simulink model "Lab4_1simulink"  (R2024b)
settings: Solver=ode45  StartTime=0.0  StopTime=t_sim  MaxStep=0.01*Ts  MinStep=0.001*Ts  RelTol=1e-3
values from neighbouring files (symbols this model uses):
  C = [1 0]    [Lab_Practice_4_1.m]
  K = dlqr(Ad, Bd, Q,R)    [Lab_Practice_4_1.m]
  Ts = 0.05    [Lab_Practice_4_1.m]
  x0 = [0.8;0]    [Lab_Practice_4_1.m]
libraries: cstblocks x1
settings Model: Creator=filoz  LastModifiedBy=filoz
settings SolverCC: InitialStep=0.001*Ts

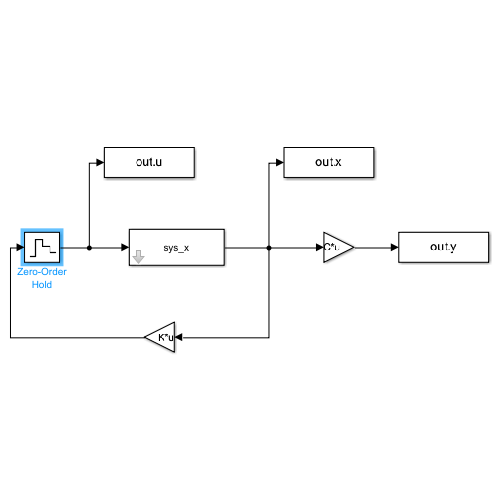
[thumbnail: Simulink's stored preview of the top-level diagram]
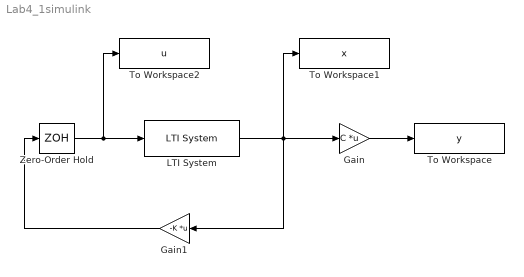
== system Lab4_1simulink ==
  Gain : Gain  Gain=C  Multiplication=Matrix(K*u)
  Gain1 : Gain  Gain=-K  Multiplication=Matrix(K*u)
  LTI System : cstblocks/LTI System  sys=sys_x  IC=[x0]  PadeOrder=0
  To Workspace : ToWorkspace  VariableName=y  SaveFormat=Timeseries  SampleTime=0.01*Ts
  To Workspace1 : ToWorkspace  VariableName=x  SaveFormat=Timeseries  SampleTime=0.01*Ts
  To Workspace2 : ToWorkspace  VariableName=u  SaveFormat=Timeseries  SampleTime=0.01*Ts
  Zero-Order Hold : ZeroOrderHold  SampleTime=Ts
  wires:
  LTI System/1 -> Gain1/1, To Workspace1/1, Gain/1
  Gain/1 -> To Workspace/1
  Zero-Order Hold/1 -> To Workspace2/1, LTI System/1
  Gain1/1 -> Zero-Order Hold/1
